simulink model "old_old"  (R2023b)
settings: Solver=FixedStepAuto  StartTime=StartTime  StopTime=34  RelTol=1e-3
values from neighbouring files (symbols this model uses):
  current_height = 0.0    (= 0)    [wrapper_for_simulink.m]
  current_pitch = 0.0    (= 0)    [wrapper_for_simulink.m]
  current_vel = 0.0    (= 0)    [wrapper_for_simulink.m]
  extension_length = 0.0    (= 0)    [wrapper_for_simulink.m]
undefined symbols (not defined in the file or in its folder): HDBK, Light, magnitude, MIL, STD
libraries: aerolibwind2 x3, aerolibasang x2, aerolibatmos2 x1
settings Model: Creator=User  LastModifiedBy=User
settings DataIOCC: ReturnWorkspaceOutputsName=tp3ca22a37_fc90_43f8_8ebe_8c0e39ad763e
settings DebuggingCC: ArtificialAlgebraicLoopMsg=none

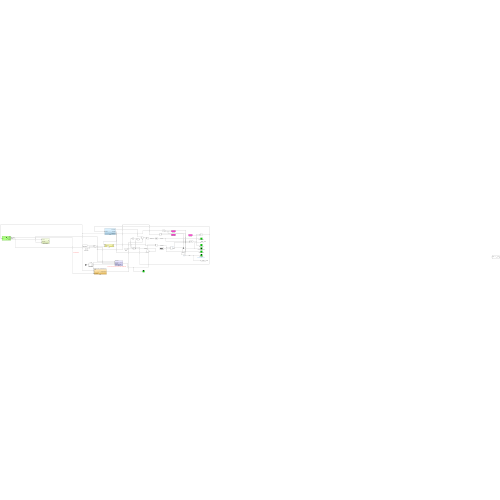
[thumbnail: Simulink's stored preview of the top-level diagram]
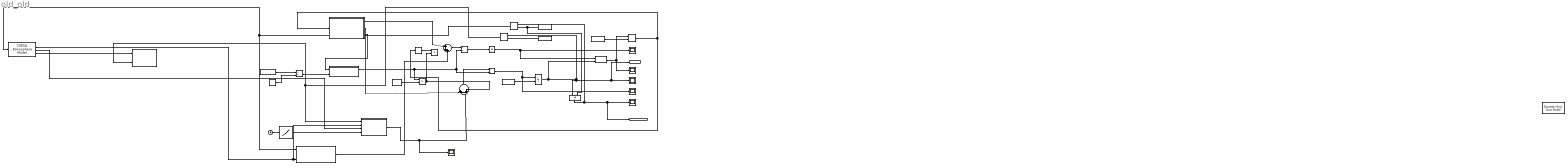
== system old_old ==
  note: ignore everything after v = 0
  note: need to figure out how the wind parameters here
  note: why is this so high???
  note: drag is too high rn at high mach, will need to wait for better drag curve
  " m(t)" : Subsystem
  Atan2 : Trigonometry  Operator=atan2
  COESA Atmosphere Model : aerolibatmos2/COESA Atmosphere Model  units=Metric (MKS)  spec=MIL-STD-210C  model=Profile  profile_var=Low temperature  profile_percent=10%  profile_alt=5 km (16404 ft)  envelope_var=High temperature  envelope_percent=1%  action=Warning
  Clock : Clock
  Delay1 : Delay  DelayLength=1  InitialConditionSource=Input port
      settings: InputPortMap=u0,p4
  Delay2 : Delay  DelayLength=1  InitialConditionSource=Input port
      settings: InputPortMap=u0,p4
  Delay3 : Delay  DelayLength=1  InitialConditionSource=Input port
      settings: InputPortMap=u0,p4
  Discrete Wind Gust Model : aerolibwind2/Discrete Wind Gust Model  units=Metric (MKS)  Gx=on  Gy=on  Gz=on  t_0=5  d_m=[120 120 80]  v_m=[3.5 3.5 3.0]
  Divide : Product  Inputs=*/
  Divide1 : Product  Inputs=*/
  Divide2 : Product  Inputs=*/
  Dynamic Pressure : Subsystem
  Extension Plan : Lookup_n-D  NumberOfTableDimensions=1  BreakpointsForDimension1=[0 4.99 5 5.01 5.011 6]  Table=[0 0 extension_length 0.99*extension_length 0 0]  InternalRulePriority=Speed  RndMeth=Simplest
  Flight path angle : Scope
  Integrator : Integrator  InitialConditionSource=external
  Integrator1 : Integrator  InitialConditionSource=external
  Integrator2 : Integrator
  Product1 : Product
  Product2 : Product
  Scope2 : Scope
  Sin : Trigonometry
  Sum : Sum  Inputs=|+--+-
  Sum1 : Sum  Inputs=|+++
  WIND : Subsystem
  current height : Constant  Value=current_height
  current pitch : Constant  Value=current_pitch
  current vel : Constant  Value=current_vel
  current velocity : Constant  Value=current_vel
  drag : Subsystem
  gravity g : Constant  Value=9.80665
  horizontal distance : Scope
  propellant mass : Constant  Value=5.07
  thrust : Subsystem
  total impulse : Constant  Value=9976.7
  vertical acceleration : Scope
  vertical height : Scope
  vertical velocity in earth ref : Scope
  Out1 : Outport  SignalName=height
  Out2 : Outport  Port=2  SignalName=velocity
  wires:
  Integrator1/1 -> Atan2/2, Integrator/1, Out2/1, vertical velocity in earth ref/1, Delay2/1  "velocity"
  COESA Atmosphere Model/2 -> drag/2(speed of sound), WIND/3(speed of sound)  "speed of sound"
  Sum/1 -> Divide1/1
  thrust/2(vertical thrust) -> Sum/1
  Delay1/1 -> Sin/1, thrust/1(pitch angle)
  drag/1(Drag Force) -> Scope2/1, Sum/3
  Delay2/1 -> drag/1(velocity vector), Dynamic Pressure/2(velocity signal)
  current velocity/1 -> Delay2/2
  current pitch/1 -> Delay1/2
  COESA Atmosphere Model/4 -> Dynamic Pressure/1(Air Density)
  " m(t)"/1(m(t)) -> Product1/1, Divide1/2, Divide2/2
  thrust/3(magnitude of T) -> " m(t)"/1(thrust)
  Integrator/1 -> Delay3/1, Out1/1, vertical height/1  "height"
  gravity g/1 -> Product1/2
  total impulse/1 -> Divide/1
  propellant mass/1 -> Divide/2
  Divide/1 -> " m(t)"/2(exhaust velocity)
  Divide1/1 -> vertical acceleration/1, Integrator1/1  "vertical accel"
  Atan2/1 -> Delay1/1, Flight path angle/1
  Delay3/1 -> WIND/1(Altitude), COESA Atmosphere Model/1
  Sum1/1 -> Divide2/1  "Fx"
  WIND/1(wind force u direction) -> Sum1/3
  Integrator2/1 -> horizontal distance/1, Atan2/1  "horizontal vel"
  Divide2/1 -> Integrator2/1  "horizontal accel"
  Product1/1 -> Sum/5, Product2/2  "gravitational"
  Sin/1 -> Product2/1
  thrust/1(horizontal thrust) -> Sum1/1
  Clock/1 -> Extension Plan/1
  Extension Plan/1 -> drag/4(Airbrakes extension plan)
  current vel/1 -> Integrator1/2
  current height/1 -> Delay3/2, Integrator/2
  COESA Atmosphere Model/3 -> drag/3(pressure(Pa))  "pressure"

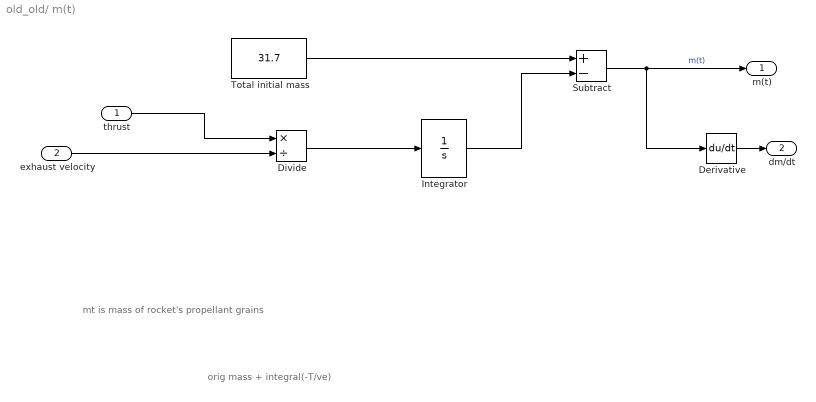
== system old_old/ m(t) ==
  note: orig mass + integral(-T/ve)
  note: mt is mass of rocket's propellant grains
  thrust : Inport
  exhaust velocity : Inport  Port=2
  Derivative : Derivative
  Divide : Product  Inputs=*/
  Integrator : Integrator
  Subtract : Sum  Inputs=+-
  Total initial mass : Constant  Value=31.7
  m(t) : Outport
  dm/dt : Outport  Port=2
  wires:
  Total initial mass/1 -> Subtract/1
  Subtract/1 -> Derivative/1, m(t)/1  "m(t)"
  thrust/1 -> Divide/1
  exhaust velocity/1 -> Divide/2
  Divide/1 -> Integrator/1
  Integrator/1 -> Subtract/2
  Derivative/1 -> dm/dt/1

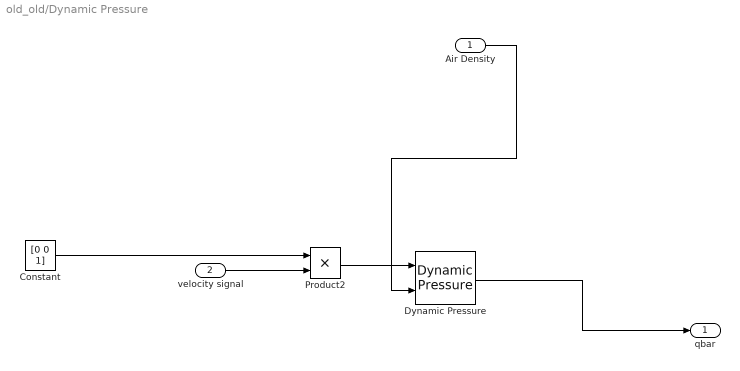
== system old_old/Dynamic Pressure ==
  Air Density : Inport
  velocity signal : Inport  Port=2
  Constant : Constant  Value=[0 0 1]  VectorParams1D=off
  Dynamic Pressure : aerolibasang/Dynamic Pressure
  Product2 : Product
  qbar : Outport
  wires:
  Product2/1 -> Dynamic Pressure/1
  Constant/1 -> Product2/1
  Dynamic Pressure/1 -> qbar/1
  Air Density/1 -> Dynamic Pressure/2
  velocity signal/1 -> Product2/2

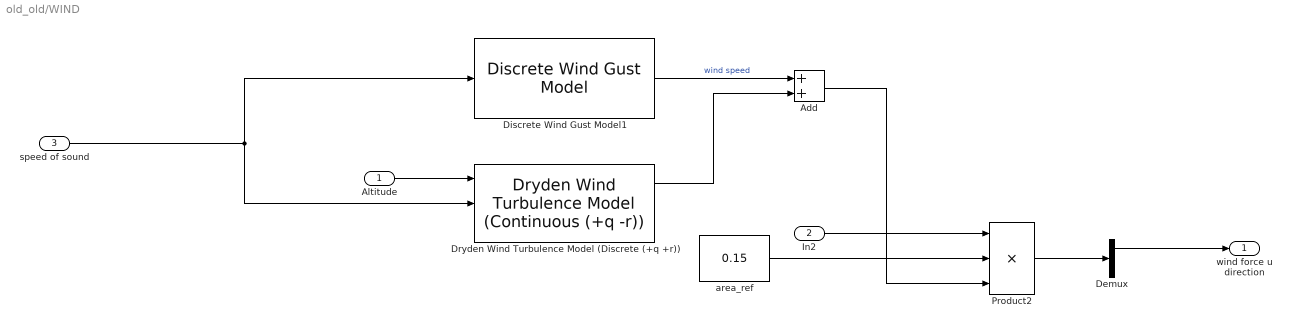
== system old_old/WIND ==
  Altitude : Inport
  In2 : Inport  Port=2
  speed of sound : Inport  Port=3
  Add : Sum
  Demux : Demux  Outputs=3
  Discrete Wind Gust Model1 : aerolibwind2/Discrete Wind Gust Model  units=Metric (MKS)  Gx=on  Gy=on  Gz=on  t_0=0  d_m=[50 80 50]  v_m=[1 2 3.0]
  Dryden Wind Turbulence Model (Discrete (+q +r)) : aerolibwind2/Dryden Wind Turbulence Model  (Continuous (+q -r))  units=Metric (MKS)  spec=MIL-HDBK-1797B  model=Discrete Dryden (+q +r)  W20=5  Wdeg=10  TurbProb=10^-2 - Light  L_high=533.4  Wingspan=10  ts=0.1  Seed=[23341 23342 23343 23344]  T_on=on
      settings: LibrarySourceBlock=|
      | aerolibwind2/Dryden Wind Turbulence Model
      | (Discrete (+q +r))
  Product2 : Product  Inputs=3
  area_ref : Constant  Value=0.15
  wind force u direction : Outport
  wires:
  In2/1 -> Product2/1
  area_ref/1 -> Product2/2
  Dryden Wind Turbulence Model (Discrete (+q +r))/1 -> Add/2
  speed of sound/1 -> Discrete Wind Gust Model1/1, Dryden Wind Turbulence Model (Discrete (+q +r))/2
  Product2/1 -> Demux/1
  Altitude/1 -> Dryden Wind Turbulence Model (Discrete (+q +r))/1
  Discrete Wind Gust Model1/1 -> Add/1  "wind speed"
  Add/1 -> Product2/3
  Demux/1 -> wind force u direction/1

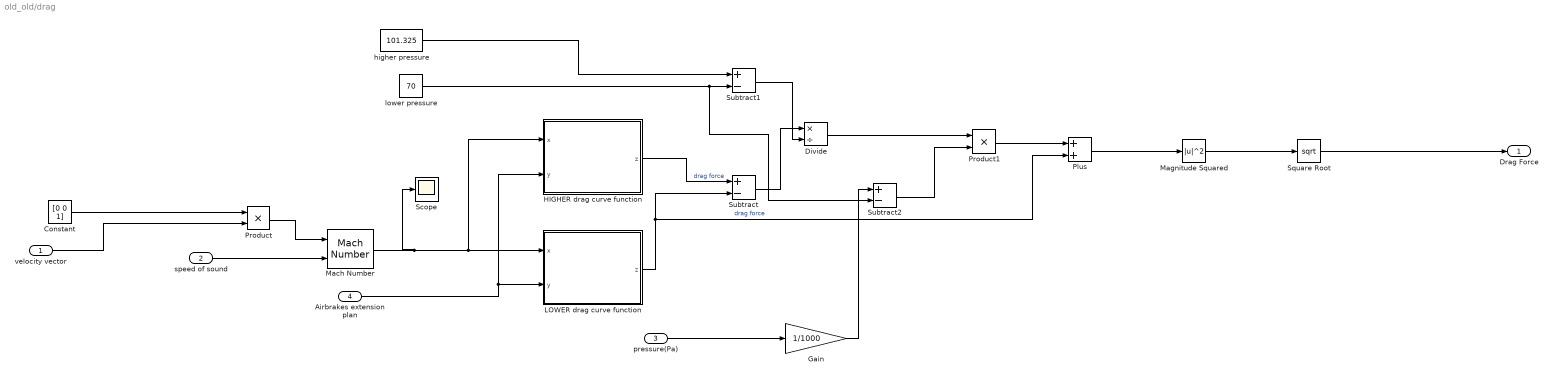
== system old_old/drag ==
  velocity vector : Inport
  speed of sound : Inport  Port=2
  pressure(Pa) : Inport  Port=3
  Airbrakes extension plan : Inport  Port=4
  Constant : Constant  Value=[0 0 1]  VectorParams1D=off
  Divide : Product  Inputs=*/
  Gain : Gain  Gain=1/1000
  HIGHER drag curve function : MATLAB Function  TreatAsAtomicUnit=on
  LOWER drag curve function : MATLAB Function  TreatAsAtomicUnit=on
  Mach Number : aerolibasang/Mach Number
  Magnitude Squared : Math  Operator=magnitude^2
  Plus : Sum
  Product : Product
  Product1 : Product
  Scope : Scope
  Square Root : Sqrt
  Subtract : Sum  Inputs=+-
  Subtract1 : Sum  Inputs=+-
  Subtract2 : Sum  Inputs=+-
  higher pressure : Constant  Value=101.325
  lower pressure : Constant  Value=70
  Drag Force : Outport
  wires:
  higher pressure/1 -> Subtract1/1
  Subtract/1 -> Divide/1
  velocity vector/1 -> Product/2
  Mach Number/1 -> Scope/1, HIGHER drag curve function/1(x), LOWER drag curve function/1(x)
  Gain/1 -> Subtract2/1
  Divide/1 -> Product1/1
  Subtract1/1 -> Divide/2
  Product1/1 -> Plus/1
  pressure(Pa)/1 -> Gain/1
  Plus/1 -> Magnitude Squared/1
  lower pressure/1 -> Subtract2/2, Subtract1/2
  Subtract2/1 -> Product1/2
  Magnitude Squared/1 -> Square Root/1
  LOWER drag curve function/1(z) -> Plus/2, Subtract/2  "drag force"
  Square Root/1 -> Drag Force/1
  speed of sound/1 -> Mach Number/2
  HIGHER drag curve function/1(z) -> Subtract/1  "drag force"
  Product/1 -> Mach Number/1
  Airbrakes extension plan/1 -> HIGHER drag curve function/2(y), LOWER drag curve function/2(y)
  Constant/1 -> Product/1

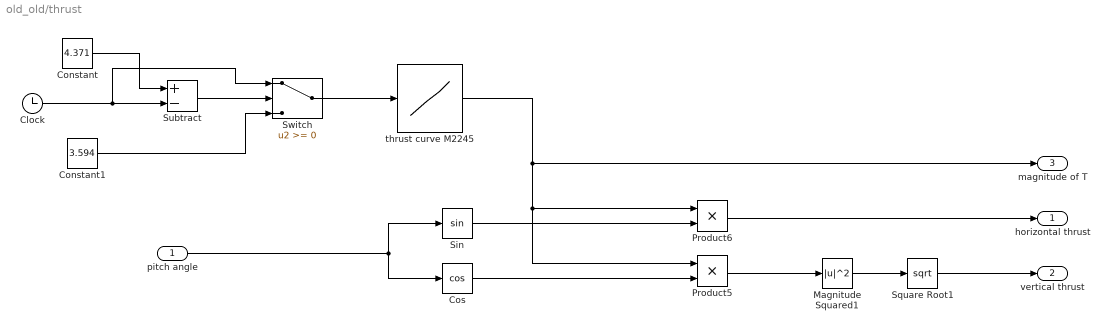
== system old_old/thrust ==
  pitch angle : Inport
  Clock : Clock
  Constant : Constant  Value=4.371
  Constant1 : Constant  Value=3.594
  Cos : Trigonometry  Operator=cos
  Magnitude Squared1 : Math  Operator=magnitude^2
  Product5 : Product
  Product6 : Product
  Sin : Trigonometry
  Square Root1 : Sqrt
  Subtract : Sum  Inputs=+-
  Switch : Switch  SaturateOnIntegerOverflow=off  InputSameDT=off
  thrust curve M2245 : Lookup_n-D  NumberOfTableDimensions=1  BreakpointsForDimension1=|  BreakpointsForDimension2=[1:3]  Table=|  InternalRulePriority=Speed  RndMeth=Simplest
      BreakpointsForDimension1=|
      | [0.043
      | 0.136
      | 1.393
      | 2.168
      | 2.708
      | 2.837
      | 3.152
      | 3.397
      | 3.878
      | 4.371]
      Table=|
      | [3045.655
      | 2629.813
      | 3003.3
      | 3007.151
      | 2972.497
      | 2883.938
      | 1955.996
      | 1409.241
      | 562.156
      | 0]
  horizontal thrust : Outport
  vertical thrust : Outport  Port=2
  magnitude of T : Outport  Port=3
  wires:
  Clock/1 -> Switch/1, Subtract/2
  thrust curve M2245/1 -> Product6/1, Product5/1, magnitude of T/1
  Cos/1 -> Product5/2
  Sin/1 -> Product6/2
  pitch angle/1 -> Sin/1, Cos/1
  Product5/1 -> Magnitude Squared1/1
  Subtract/1 -> Switch/2
  Constant/1 -> Subtract/1
  Switch/1 -> thrust curve M2245/1
  Constant1/1 -> Switch/3
  Product6/1 -> horizontal thrust/1
  Magnitude Squared1/1 -> Square Root1/1
  Square Root1/1 -> vertical thrust/1

== matlab function old_old/drag/LOWER drag curve function ==
  data: x input; z output; y input
function z = fcn(x, y)
%x is mach number, y is extension in m
z = 68.2243 -668.2799*x -1.1397e+03*y + 1.3993e+03*x^2 + 1.3374e+04*x*y + 8.1616e+04 *y^2 -349.7704*x^3 -3.3397e+04*x^2*y + 6.5648e+05*x*y^2 -7.5125e+06*y^3

== matlab function old_old/drag/HIGHER drag curve function ==
  data: x input; z output; y input
function z = fcn(x, y)
%x is mach number, y is extension in m
z = 23.6982 -123.4344*x - 2.5545e+03*y + 402.1042*x^2 + 9.1165e+03*x*y + 4.4646e+04*y^2
